simulink model "p3"  (R2019b)
settings: Solver=VariableStepAuto  StartTime=0.0  StopTime=100  RelTol=1e-3
values from neighbouring files (symbols this model uses):
  A = [ 0             0         1              0 ... (first row only)    [p3.m]
  B = [0; 0; 1; 0]    [p3.m]
  C = [1 0 0 0]    [p3.m]
  Kr = G2-W1*C'*Qy    [p3.m]
  Kw = K_(:,nx+1:nx+ny)    [p3.m]
  Kx = Khat(:,1:nx)    [p3.m]
  r = 10    [p3.m]
undefined symbols (not defined in the file or in its folder): X0
settings Model: Creator=samel  LastModifiedBy=sharathchandra
settings DataIOCC: ReturnWorkspaceOutputs=off
settings DebuggingCC: ArithmeticOperatorsInVariantConditions=warning
settings SFSimCC: CustomCodeUndefinedFunction=UseInterfaceOnly

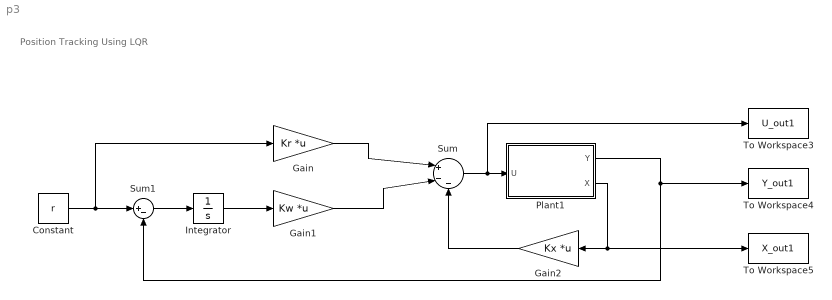
== system p3 ==
  note: Position Tracking Using LQR
  Constant : Constant  Value=r
  Gain : Gain  Gain=Kr  Multiplication=Matrix(K*u)
  Gain1 : Gain  Gain=Kw  Multiplication=Matrix(K*u)
  Gain2 : Gain  Gain=Kx  Multiplication=Matrix(K*u)
  Integrator : Integrator
  Plant1 : Subsystem
  Sum : Sum  Inputs=|+--
  Sum1 : Sum  Inputs=|+-
  To Workspace3 : ToWorkspace  VariableName=U_out1  SampleTime=-1
      settings: Save2DSignal=2-D array (concatenate along first dimension)
  To Workspace4 : ToWorkspace  VariableName=Y_out1  SampleTime=-1
      settings: Save2DSignal=2-D array (concatenate along first dimension)
  To Workspace5 : ToWorkspace  VariableName=X_out1  SampleTime=-1
      settings: Save2DSignal=2-D array (concatenate along first dimension)
  wires:
  Gain/1 -> Sum/1
  Gain1/1 -> Sum/2
  Plant1/2(X) -> To Workspace5/1, Gain2/1
  Gain2/1 -> Sum/3
  Constant/1 -> Gain/1, Sum1/1
  Plant1/1(Y) -> Sum1/2, To Workspace4/1
  Sum1/1 -> Integrator/1
  Integrator/1 -> Gain1/1
  Sum/1 -> To Workspace3/1, Plant1/1(U)

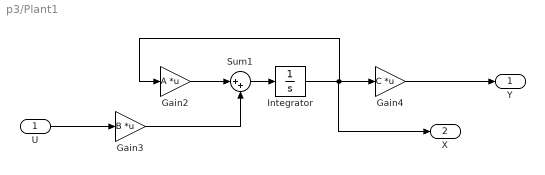
== system p3/Plant1 ==
  U : Inport
  Gain2 : Gain  Gain=A  Multiplication=Matrix(K*u)
  Gain3 : Gain  Gain=B  Multiplication=Matrix(K*u)
  Gain4 : Gain  Gain=C  Multiplication=Matrix(K*u)
  Integrator : Integrator  InitialCondition=X0
  Sum1 : Sum  Inputs=|++
  Y : Outport  VectorParamsAs1DForOutWhenUnconnected=off
  X : Outport  Port=2  VectorParamsAs1DForOutWhenUnconnected=off
  wires:
  Gain2/1 -> Sum1/1
  Gain4/1 -> Y/1
  Integrator/1 -> X/1, Gain2/1, Gain4/1
  Sum1/1 -> Integrator/1
  Gain3/1 -> Sum1/2
  U/1 -> Gain3/1
